simulink model "kiem_chung_con_lac_r2021b"  (R2021b)
settings: Solver=ode23  StartTime=0.0  StopTime=2.5  RelTol=1e-3
undefined symbols (not defined in the file): G1, G2, Kdc, Kic, Kpc
settings Model: Creator=datng  LastModifiedBy=datng
settings DebuggingCC: UnconnectedInputMsg=none  UnconnectedOutputMsg=none  UnconnectedLineMsg=none
settings ModelReferenceCC: EnableRefExpFcnMdlSchedulingChecks=off
settings RTWCC: GPUComputeCapability=5.0  DLArmComputeVersion=20.02.1
settings ConfigComp: CovBoundaryAbsTol=1.0e-5

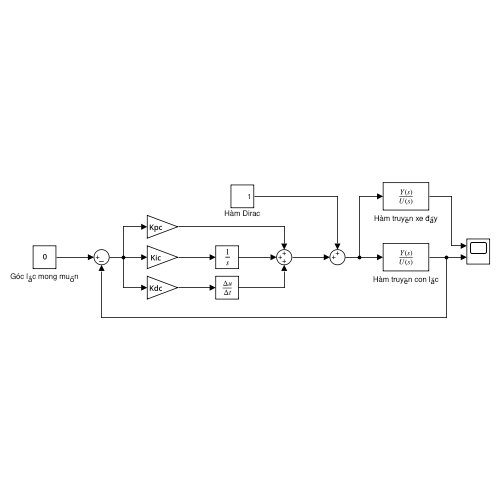
[thumbnail: Simulink's stored preview of the top-level diagram]
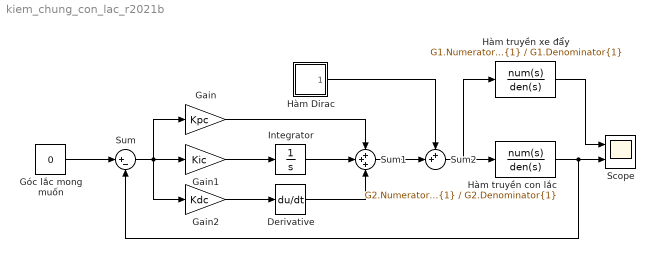
== system kiem_chung_con_lac_r2021b ==
  Derivative : Derivative  CoefficientInTFapproximation=0
  Gain : Gain  Gain=Kpc
  Gain1 : Gain  Gain=Kic
  Gain2 : Gain  Gain=Kdc
  Góc lắc mong muốn : Constant  Value=0
  Hàm Dirac : Subsystem
  Hàm truyền con lắc : TransferFcn  Numerator=G2.Numerator{1}  Denominator=G2.Denominator{1}
  Hàm truyền xe đẩy : TransferFcn  Numerator=G1.Numerator{1}  Denominator=G1.Denominator{1}
  Integrator : Integrator
  Scope : Scope  NumInputPorts=2
  Sum : Sum  Inputs=|+-
  Sum1 : Sum  Inputs=+++
  Sum2 : Sum  Inputs=++|
  wires:
  Góc lắc mong muốn/1 -> Sum/1
  Sum/1 -> Gain/1, Gain2/1, Gain1/1
  Gain1/1 -> Integrator/1
  Integrator/1 -> Sum1/2
  Derivative/1 -> Sum1/3
  Gain2/1 -> Derivative/1
  Gain/1 -> Sum1/1
  Sum1/1 -> Sum2/2
  Hàm Dirac/1(1) -> Sum2/1
  Sum2/1 -> Hàm truyền xe đẩy/1, Hàm truyền con lắc/1
  Hàm truyền con lắc/1 -> Scope/2, Sum/2
  Hàm truyền xe đẩy/1 -> Scope/1

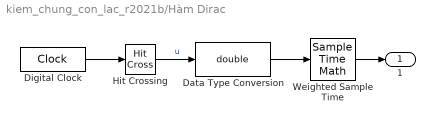
== system kiem_chung_con_lac_r2021b/Hàm Dirac ==
  Data Type Conversion : DataTypeConversion  OutDataTypeStr=double
  Digital Clock : DigitalClock  SampleTime=0.001
  Hit Crossing : HitCross
  Weighted Sample Time : SampleTimeMath  TsampMathOp=/
  1 : Outport
  wires:
  Digital Clock/1 -> Hit Crossing/1
  Hit Crossing/1 -> Data Type Conversion/1  "u"
  Data Type Conversion/1 -> Weighted Sample Time/1
  Weighted Sample Time/1 -> 1/1
